simulink subsystem "Multiple_ECG_Signal_QRS_Detector"  (R2021a)
settings: Solver=VariableStepAuto  StartTime=0.0  StopTime=10.0  RelTol=1e-3
libraries: QRS_Detector_Library x8
Description:
  | This subsytem is a nontunable QRS detector based on the Pan-Tompkin Algorithm. This subsystem
  | takes a raw ecg signal and performs filtering on the signal, as well as signal processing to identify
  | the QRS wave of the ECG signal. The outputs of this subystem are the following: post bandpass,
  | post derivative, post squaring, post moving average, post threshold 2, post threshold 1,
  | and finally the QRS detection output.
settings Model: Creator=wallyproenza  LastModifiedBy=wallyproenza

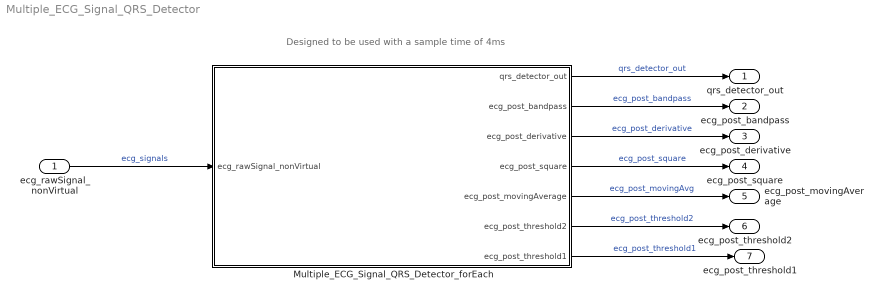
== system Multiple_ECG_Signal_QRS_Detector ==
  note: Designed to be used with a sample time of 4ms
  ecg_rawSignal_nonVirtual : Inport
  Multiple_ECG_Signal_QRS_Detector_forEach : Subsystem  TreatAsAtomicUnit=on
  qrs_detector_out : Outport
  ecg_post_bandpass : Outport  Port=2
  ecg_post_derivative : Outport  Port=3
  ecg_post_square : Outport  Port=4
  ecg_post_movingAverage : Outport  Port=5
  ecg_post_threshold2 : Outport  Port=6
  ecg_post_threshold1 : Outport  Port=7
  wires:
  Multiple_ECG_Signal_QRS_Detector_forEach/4(ecg_post_square) -> ecg_post_square/1  "ecg_post_square"
  Multiple_ECG_Signal_QRS_Detector_forEach/7(ecg_post_threshold1) -> ecg_post_threshold1/1  "ecg_post_threshold1"
  Multiple_ECG_Signal_QRS_Detector_forEach/3(ecg_post_derivative) -> ecg_post_derivative/1  "ecg_post_derivative"
  Multiple_ECG_Signal_QRS_Detector_forEach/6(ecg_post_threshold2) -> ecg_post_threshold2/1  "ecg_post_threshold2"
  Multiple_ECG_Signal_QRS_Detector_forEach/1(qrs_detector_out) -> qrs_detector_out/1  "qrs_detector_out"
  Multiple_ECG_Signal_QRS_Detector_forEach/2(ecg_post_bandpass) -> ecg_post_bandpass/1  "ecg_post_bandpass"
  Multiple_ECG_Signal_QRS_Detector_forEach/5(ecg_post_movingAverage) -> ecg_post_movingAverage/1  "ecg_post_movingAvg"
  ecg_rawSignal_nonVirtual/1 -> Multiple_ECG_Signal_QRS_Detector_forEach/1(ecg_rawSignal_nonVirtual)  "ecg_signals"

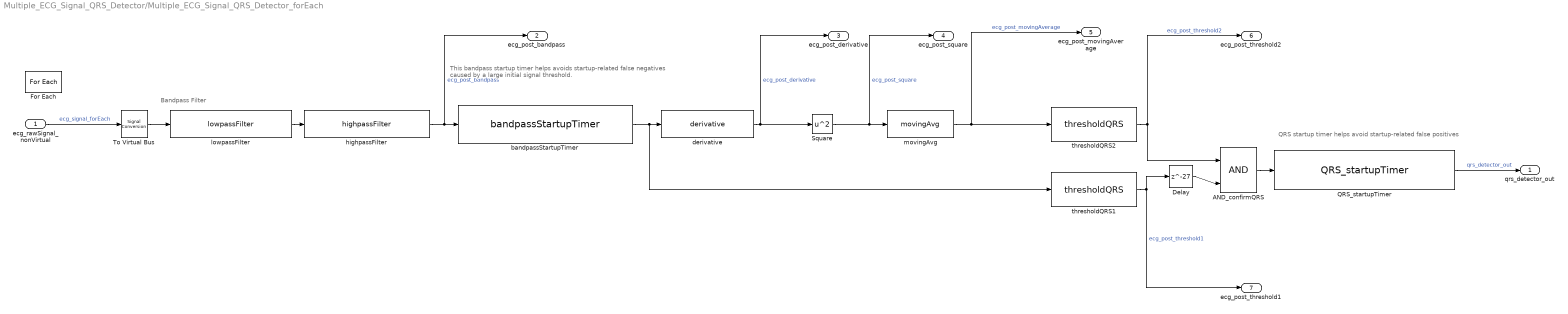
== system Multiple_ECG_Signal_QRS_Detector/Multiple_ECG_Signal_QRS_Detector_forEach ==
  note: QRS startup timer helps avoid startup-related false positives
  note: Bandpass Filter
  note: This bandpass startup timer helps avoids startup-related false negatives
      | caused by a large initial signal threshold.
  ecg_rawSignal_nonVirtual : Inport  Partition=on  PartitionDimension=1  PartitionWidth=1  PartitionOffset=0
  AND_confirmQRS : Logic  IconShape=distinctive  AllPortsSameDT=off  OutDataTypeStr=boolean
  Delay : Delay  DelayLength=27  InitialCondition=0
  For Each : ForEach  DisableCoverage=on
  QRS_startupTimer : QRS_Detector_Library/QRS_startupTimer  SystemSampleTime=-1  VariantActivationTime=update diagram  Latency=0  AutoFrameSizeCalculation=off
  Square : Math  Operator=square  SaturateOnIntegerOverflow=on
  To Virtual Bus : SignalConversion  ConversionOutput=Virtual bus  OverrideOpt=off
  bandpassStartupTimer : QRS_Detector_Library/bandpassStartupTimer  SystemSampleTime=-1  VariantActivationTime=update diagram  Latency=0  AutoFrameSizeCalculation=off
  derivative : QRS_Detector_Library/derivative  SystemSampleTime=-1  VariantActivationTime=update diagram  Latency=0  AutoFrameSizeCalculation=off
  highpassFilter : QRS_Detector_Library/highpassFilter  SystemSampleTime=-1  VariantActivationTime=update diagram  Latency=0  AutoFrameSizeCalculation=off
  lowpassFilter : QRS_Detector_Library/lowpassFilter  SystemSampleTime=-1  VariantActivationTime=update diagram  Latency=0  AutoFrameSizeCalculation=off
  movingAvg : QRS_Detector_Library/movingAvg  SystemSampleTime=-1  VariantActivationTime=update diagram  Latency=0  AutoFrameSizeCalculation=off
  thresholdQRS1 : QRS_Detector_Library/thresholdQRS  SystemSampleTime=-1  VariantActivationTime=update diagram  Latency=0  AutoFrameSizeCalculation=off
  thresholdQRS2 : QRS_Detector_Library/thresholdQRS  SystemSampleTime=-1  VariantActivationTime=update diagram  Latency=0  AutoFrameSizeCalculation=off
  qrs_detector_out : Outport  ConcatenationDimension=1
  ecg_post_bandpass : Outport  Port=2  ConcatenationDimension=1
  ecg_post_derivative : Outport  Port=3  ConcatenationDimension=1
  ecg_post_square : Outport  Port=4  ConcatenationDimension=1
  ecg_post_movingAverage : Outport  Port=5  ConcatenationDimension=1
  ecg_post_threshold2 : Outport  Port=6  ConcatenationDimension=1
  ecg_post_threshold1 : Outport  Port=7  ConcatenationDimension=1
  wires:
  Square/1 -> movingAvg/1, ecg_post_square/1  "ecg_post_square"
  QRS_startupTimer/1 -> qrs_detector_out/1  "qrs_detector_out"
  AND_confirmQRS/1 -> QRS_startupTimer/1
  bandpassStartupTimer/1 -> derivative/1, thresholdQRS1/1
  thresholdQRS1/1 -> ecg_post_threshold1/1, Delay/1  "ecg_post_threshold1"
  thresholdQRS2/1 -> ecg_post_threshold2/1, AND_confirmQRS/1  "ecg_post_threshold2"
  highpassFilter/1 -> ecg_post_bandpass/1, bandpassStartupTimer/1  "ecg_post_bandpass"
  lowpassFilter/1 -> highpassFilter/1
  ecg_rawSignal_nonVirtual/1 -> To Virtual Bus/1  "ecg_signal_forEach"
  To Virtual Bus/1 -> lowpassFilter/1
  Delay/1 -> AND_confirmQRS/2
  derivative/1 -> ecg_post_derivative/1, Square/1  "ecg_post_derivative"
  movingAvg/1 -> ecg_post_movingAverage/1, thresholdQRS2/1  "ecg_post_movingAverage"
